simulink model "CtrPlatform_gravity_compensation"  (Simulink 7.9)
settings: Solver=ode3  StartTime=0.0  StopTime=4  FixedStep=Ts  RelTol=1e-3
InitFcn:
  | eval('Config')
StopFcn:
  | eval('tu')
values from neighbouring files (symbols this model uses):
  A = [a1 a2 a3 a4 a5 a6]/180*pi    [Config.m]    (also in CtrPlatformCfg.m)
  a2 = 0    [Config.m]    (also in CtrPlatformCfg.m)
  a3 = 0    [Config.m]    (also in CtrPlatformCfg.m)
  a4 = 0    [Config.m]    (also in CtrPlatformCfg.m)
  a5 = 90    [Config.m]    (also in CtrPlatformCfg.m)
  a6 = 0    [Config.m]    (also in CtrPlatformCfg.m)
  Cen = Cen(:)'    [Config.m]    (also in CtrPlatformCfg.m; DynEulerTest.m = Cen'; EfDynCAD.m = [cen1,cen2,cen3,cen4,cen5,cen6]')
  CurPulseFreq = 0.25*2*pi    (= 1.57079632679)    [Config.m]    (also in CtrPlatformCfg.m)
  Deg2Rad = pi/180    (= 0.0174532925199)    [Config.m]    (also in CtrPlatformCfg.m)
  DisturbSelect = 2    [Config.m]    (also in CtrPlatformCfg.m)
  DynTrjMode = 3    [Config.m]    (also in CtrPlatformCfg.m = 1)
  FbDisturbSelect = 2    [Config.m]    (also in CtrPlatformCfg.m)
  freq = tvel/radius    (= 1)    [Config.m]    (also in CtrPlatformCfg.m)
  Gravity = 9.8    [Config.m]    (also in CtrPlatformCfg.m)
  Ie1 = in1(:)'    [Config.m]    (also in CtrPlatformCfg.m; DynEulerTest.m = in1(:); EfDynCAD.m = in1(:))
  Ie2 = in2(:)'    [Config.m]    (also in CtrPlatformCfg.m; DynEulerTest.m = in2(:); EfDynCAD.m = in2(:))
  Ie3 = in3(:)'    [Config.m]    (also in CtrPlatformCfg.m; DynEulerTest.m = in3(:); EfDynCAD.m = in3(:))
  Ie4 = in4(:)'    [Config.m]    (also in CtrPlatformCfg.m; DynEulerTest.m = in4(:); EfDynCAD.m = in4(:))
  Ie5 = in5(:)'    [Config.m]    (also in CtrPlatformCfg.m; DynEulerTest.m = in5(:); EfDynCAD.m = in5(:))
  Ie6 = in6(:)'    [Config.m]    (also in CtrPlatformCfg.m; DynEulerTest.m = in6(:); EfDynCAD.m = in6(:))
  in1 = [5.2954 -0.2565 -0.6366;-0.2565 4.7000 0.2830;-0.6366 0.2829 5.8635]    [Config.m]    (also in CtrPlatformCfg.m; DynEulerTest.m; EfDynCAD.m = [0.54  -0.01 0.23)
  in2 = [5.8840 0.0072 0.0135;0.0072 6.0178 -0.1907;0.0135 -0.1907 0.3374]    [Config.m]    (also in CtrPlatformCfg.m; DynEulerTest.m; EfDynCAD.m = (R_x*R_z)*in2*(R_x*R_z)')
  in3 = [1.8201 -0.2274 -0.3112;-0.2274 2.2537 -0.1441;-0.3112 -0.1441 1.9485]    [Config.m]    (also in CtrPlatformCfg.m; DynEulerTest.m; EfDynCAD.m = (R_x*R_z)*in3*(R_x*R_z)')
  in4 = [0.0607 -0.0922 0;-0.0922 1.4493 0;0 0 1.4620]    [Config.m]    (also in CtrPlatformCfg.m; DynEulerTest.m = [0.0607 -0.0922 0;-0.0922 1.4493 0;0 0,1.4620]; EfDynCAD.m = (R_y*Rz)*in4*(R_y*Rz)')
  in5 = [0.0191 0.0032 0;0.0032 0.0228 0;0 0 0.0291]    [Config.m]    (also in CtrPlatformCfg.m; DynEulerTest.m; EfDynCAD.m = (R_x*R_y)*in5*(R_x*R_y)')
  in6 = [0.0012 0 0;0 0.0007 0;0 0 0.0007]    [Config.m]    (also in CtrPlatformCfg.m; DynEulerTest.m; EfDynCAD.m = (R_y*Rz)*in6*(R_y*Rz)')
  init_Endx = gd_init(1,4)    [Config.m]    (also in CtrPlatformCfg.m)
  init_Endy = gd_init(2,4)    [Config.m]    (also in CtrPlatformCfg.m)
  init_Endz = gd_init(3,4)    [Config.m]    (also in CtrPlatformCfg.m)
  init_Rot = gd_init(1:3,1:3)    [Config.m]    (also in CtrPlatformCfg.m)
  JntOffset1 = A(1)    [Config.m]    (also in CtrPlatformCfg.m)
  JntOffset2 = A(2)    [Config.m]    (also in CtrPlatformCfg.m)
  JntOffset3 = A(3)    [Config.m]    (also in CtrPlatformCfg.m)
  JntOffset4 = A(4)    [Config.m]    (also in CtrPlatformCfg.m)
  JntOffset5 = A(5)    [Config.m]    (also in CtrPlatformCfg.m)
  JntOffset6 = A(6)    [Config.m]    (also in CtrPlatformCfg.m)
  L = [l1 l2 l3 l4 l5 l6 l7 l8 l9]    [Config.m]    (also in CtrPlatformCfg.m)
  LinePTs2RadpS = 2*pi/(EncRes*Ts)./Gear    [Config.m]    (also in CtrPlatformCfg.m)
  LinePTs2Rpm = 60/(EncRes*Ts)    (= 7.32421875)    [Config.m]    (also in CtrPlatformCfg.m)
  Ma = [ma1 ma2 ma3 ma4 ma5 ma6]    [Config.m]    (also in CtrPlatformCfg.m; DynEulerTest.m = [ma1; ma2; ma3; ma4; ma5; ma6]; EfDynCAD.m = [ma1 ma2 ma3 ma4 ma5 ma6]')
  ma1 = 170.31    [Config.m]    (also in CtrPlatformCfg.m; DynEulerTest.m; EfDynCAD.m = 77.75)
  ma2 = 63.74    [Config.m]    (also in CtrPlatformCfg.m; DynEulerTest.m; EfDynCAD.m = 32.31)
  ma3 = 98.98    [Config.m]    (also in CtrPlatformCfg.m; DynEulerTest.m; EfDynCAD.m = 18.61)
  ma4 = 24.46    [Config.m]    (also in CtrPlatformCfg.m; DynEulerTest.m; EfDynCAD.m = 15.65)
  ma5 = 5.24    [Config.m]    (also in CtrPlatformCfg.m; DynEulerTest.m; EfDynCAD.m = 3.32)
  ma6 = 0.6    [Config.m]    (also in CtrPlatformCfg.m; DynEulerTest.m; EfDynCAD.m)
  PosPulseEnable = 1    [Config.m]    (also in CtrPlatformCfg.m)
  PosVelPulseGain = 500    [Config.m]    (also in CtrPlatformCfg.m)
  Rad2Line = Gear*EncRes/(2*pi)    [Config.m]    (also in CtrPlatformCfg.m)
  Rpm2LinePTs = EncRes*Ts/60    (= 0.136533333333)    [Config.m]    (also in CtrPlatformCfg.m)
  TrajSwitch = 1    [Config.m]    (also in CtrPlatformCfg.m)
  Trq2Cur = Trq2Cur./Cur2Trq    [Config.m]    (also in CtrPlatformCfg.m)
  Ts = 1/FrHz    (= 0.00025)    [Config.m]    (also in CtrPlatformCfg.m)
  Ts_Dyn = Ts    (= 0.00025)    [Config.m]    (also in CtrPlatformCfg.m)
  tvel = 120    [Config.m]    (also in CtrPlatformCfg.m)
  VelLpAxisNum = 1    [Config.m]    (also in CtrPlatformCfg.m)
  VelPulseEnable = 0    [Config.m]    (also in CtrPlatformCfg.m)
  VelPulseGain = 500    [Config.m]    (also in CtrPlatformCfg.m)
  Volt2Trq = Volt2Trq./Trq2Cur    [Config.m]    (also in CtrPlatformCfg.m)
undefined symbols (not defined in the file or in its folder): a1, DiscIntNeverNeededParam, RobotAxis
libraries: simulink x55, mblibv1 x35, powerlib_extras x9, commnoisgen2 x2
(part 4 of 4)

== system CtrPlatform_gravity_compensation/Dynamics/TrjSource/Position Loop Tunning/Axis4 ==
  AbsEnc4 : Constant  Value=JntOffset4
  Discrete Derivative : simulink/Discrete/Discrete Derivative  gainval=1.0  ICPrevScaledInput=0.0  InputProcessing=Inherited  OutMin=[]  OutMax=[]  OutDataType=sfix(16)  OutScaling=2^-10  DoSatur=off
  Discrete-Time Integrator : DiscreteIntegrator  SampleTime=-1  ICPrevOutput=DiscIntNeverNeededParam  ICPrevScaledInput=DiscIntNeverNeededParam
  JntOffset1 : Constant  Value=JntOffset1
  JntOffset2 : Constant  Value=JntOffset2
  JntOffset3 : Constant  Value=JntOffset3
  JntOffset5 : Constant  Value=JntOffset5
  JntOffset6 : Constant  Value=JntOffset6
  LinePTs2RadpS : Gain  Gain=LinePTs2RadpS(4)
  Mux : Mux  Inputs=6
  Mux1 : Mux  Inputs=6
  Mux2 : Mux  Inputs=6
  Sum : Sum  Inputs=++|
  Zero : Constant  Value=0
  JntPos(Rad) : Outport
  JntVel(Rad/s) : Outport  Port=2
  JntAcc(Rad/s2) : Outport  Port=3
  wires:
  LinePTs2RadpS/1 -> Mux1/4, Discrete Derivative/1, Discrete-Time Integrator/1
  Sum/1 -> Mux/4
  JntOffset1/1 -> Mux/1
  [PosVel_Pulse_Dyn] -> LinePTs2RadpS/1
  Discrete Derivative/1 -> Mux2/1
  Discrete-Time Integrator/1 -> Sum/2
  AbsEnc4/1 -> Sum/1
  JntOffset2/1 -> Mux/2
  JntOffset3/1 -> Mux/3
  JntOffset5/1 -> Mux/5
  JntOffset6/1 -> Mux/6
  Zero/1 -> Mux2/6, Mux2/5, Mux2/4, Mux2/3, Mux2/2, Mux1/6, Mux1/1, Mux1/2, Mux1/3, Mux1/5
  Mux/1 -> JntPos(Rad)/1
  Mux1/1 -> JntVel(Rad/s)/1
  Mux2/1 -> JntAcc(Rad/s2)/1

== system CtrPlatform_gravity_compensation/Dynamics/TrjSource/Position Loop Tunning/Axis5 ==
  Discrete Derivative : simulink/Discrete/Discrete Derivative  gainval=1.0  ICPrevScaledInput=0.0  InputProcessing=Inherited  OutMin=[]  OutMax=[]  OutDataType=sfix(16)  OutScaling=2^-10  DoSatur=off
  Discrete-Time Integratr : DiscreteIntegrator  SampleTime=-1  ICPrevOutput=DiscIntNeverNeededParam  ICPrevScaledInput=DiscIntNeverNeededParam
  JntOffset1 : Constant  Value=JntOffset1
  JntOffset2 : Constant  Value=JntOffset2
  JntOffset3 : Constant  Value=JntOffset3
  JntOffset4 : Constant  Value=JntOffset4
  JntOffset5 : Constant  Value=JntOffset5
  JntOffset6 : Constant  Value=JntOffset6
  LinePTs2RadpS : Gain  Gain=LinePTs2RadpS(5)
  Mux : Mux  Inputs=6
  Mux1 : Mux  Inputs=6
  Mux2 : Mux  Inputs=6
  Sum : Sum  Inputs=++|
  Zero : Constant  Value=0
  JntPos(Rad) : Outport
  JntVel(Rad/s) : Outport  Port=2
  JntAcc(Rad/s2) : Outport  Port=3
  wires:
  LinePTs2RadpS/1 -> Mux1/5, Discrete Derivative/1, Discrete-Time Integratr/1
  Discrete Derivative/1 -> Mux2/5
  Sum/1 -> Mux/5
  JntOffset1/1 -> Mux/1
  Mux2/1 -> JntAcc(Rad/s2)/1
  Mux1/1 -> JntVel(Rad/s)/1
  Mux/1 -> JntPos(Rad)/1
  Zero/1 -> Mux2/1, Mux1/1, Mux1/2, Mux1/3, Mux1/4, Mux1/6, Mux2/2, Mux2/3, Mux2/4, Mux2/6
  JntOffset6/1 -> Mux/6
  JntOffset4/1 -> Mux/4
  JntOffset3/1 -> Mux/3
  JntOffset2/1 -> Mux/2
  JntOffset5/1 -> Sum/1
  Discrete-Time Integratr/1 -> Sum/2
  [PosVel_Pulse_Dyn] -> LinePTs2RadpS/1

== system CtrPlatform_gravity_compensation/Dynamics/TrjSource/Position Loop Tunning/Axis6 ==
  Discrete Derivative : simulink/Discrete/Discrete Derivative  gainval=1.0  ICPrevScaledInput=0.0  InputProcessing=Inherited  OutMin=[]  OutMax=[]  OutDataType=sfix(16)  OutScaling=2^-10  DoSatur=off
  Discrete-Time Integrator : DiscreteIntegrator  SampleTime=-1  ICPrevOutput=DiscIntNeverNeededParam  ICPrevScaledInput=DiscIntNeverNeededParam
  JntOffset1 : Constant  Value=JntOffset1
  JntOffset2 : Constant  Value=JntOffset2
  JntOffset3 : Constant  Value=JntOffset3
  JntOffset4 : Constant  Value=JntOffset4
  JntOffset5 : Constant  Value=JntOffset5
  JntOffset6 : Constant  Value=JntOffset6
  LinePTs2RadpS : Gain  Gain=LinePTs2RadpS(6)
  Mux : Mux  Inputs=6
  Mux1 : Mux  Inputs=6
  Mux2 : Mux  Inputs=6
  Sum : Sum  Inputs=++|
  Zero : Constant  Value=0
  JntPos(Rad) : Outport
  JntVel(Rad/s) : Outport  Port=2
  JntAcc(Rad/s2) : Outport  Port=3
  wires:
  LinePTs2RadpS/1 -> Mux1/6, Discrete Derivative/1, Discrete-Time Integrator/1
  Discrete Derivative/1 -> Mux2/6
  JntOffset1/1 -> Mux/1
  Sum/1 -> Mux/6
  [PosVel_Pulse_Dyn] -> LinePTs2RadpS/1
  Discrete-Time Integrator/1 -> Sum/2
  JntOffset6/1 -> Sum/1
  JntOffset2/1 -> Mux/2
  JntOffset3/1 -> Mux/3
  JntOffset4/1 -> Mux/4
  JntOffset5/1 -> Mux/5
  Zero/1 -> Mux2/5, Mux2/4, Mux2/3, Mux2/2, Mux1/5, Mux1/4, Mux1/1, Mux1/2, Mux1/3, Mux2/1
  Mux/1 -> JntPos(Rad)/1
  Mux1/1 -> JntVel(Rad/s)/1
  Mux2/1 -> JntAcc(Rad/s2)/1

== system CtrPlatform_gravity_compensation/Dynamics/TrjSource/Velocity Loop Tunning/Axis1 ==
  Discrete Derivative : simulink/Discrete/Discrete Derivative  gainval=1.0  ICPrevScaledInput=0.0  InputProcessing=Inherited  OutMin=[]  OutMax=[]  OutDataType=sfix(16)  OutScaling=2^-10  DoSatur=off
  Discrete-Time Integrator : DiscreteIntegrator  SampleTime=-1  ICPrevOutput=DiscIntNeverNeededParam  ICPrevScaledInput=DiscIntNeverNeededParam
  JntOffset1 : Constant  Value=JntOffset1  SampleTime=Ts_Dyn
  JntOffset2 : Constant  Value=JntOffset2  SampleTime=Ts_Dyn
  JntOffset3 : Constant  Value=JntOffset3  SampleTime=Ts_Dyn
  JntOffset4 : Constant  Value=JntOffset4  SampleTime=Ts_Dyn
  JntOffset5 : Constant  Value=JntOffset5  SampleTime=Ts_Dyn
  JntOffset6 : Constant  Value=JntOffset6  SampleTime=Ts_Dyn
  LinePTs2RadpS : Gain  Gain=LinePTs2RadpS(1)
  Mux : Mux  Inputs=6
  Mux1 : Mux  Inputs=6
  Mux2 : Mux  Inputs=6
  Sum : Sum  Inputs=++|
  Zero : Constant  Value=0  SampleTime=Ts_Dyn
  JntPos(Rad) : Outport
  JntVel(Rad/s) : Outport  Port=2
  JntAcc(Rad/s2) : Outport  Port=3
  wires:
  [Vel_Pulse_Dyn] -> LinePTs2RadpS/1
  Discrete Derivative/1 -> Mux2/1
  Sum/1 -> Mux/1
  JntOffset1/1 -> Sum/1
  JntOffset2/1 -> Mux/2
  JntOffset3/1 -> Mux/3
  JntOffset4/1 -> Mux/4
  JntOffset5/1 -> Mux/5
  JntOffset6/1 -> Mux/6
  Zero/1 -> Mux2/6, Mux2/5, Mux2/4, Mux2/3, Mux2/2, Mux1/6, Mux1/5, Mux1/4, Mux1/3, Mux1/2
  Mux/1 -> JntPos(Rad)/1
  Mux1/1 -> JntVel(Rad/s)/1
  Mux2/1 -> JntAcc(Rad/s2)/1
  LinePTs2RadpS/1 -> Discrete Derivative/1, Mux1/1, Discrete-Time Integrator/1
  Discrete-Time Integrator/1 -> Sum/2

== system CtrPlatform_gravity_compensation/Dynamics/TrjSource/Velocity Loop Tunning/Axis2 ==
  Discrete Derivative : simulink/Discrete/Discrete Derivative  gainval=1.0  ICPrevScaledInput=0.0  InputProcessing=Inherited  OutMin=[]  OutMax=[]  OutDataType=sfix(16)  OutScaling=2^-10  DoSatur=off
  Discrete-Time Integrator : DiscreteIntegrator  SampleTime=-1  ICPrevOutput=DiscIntNeverNeededParam  ICPrevScaledInput=DiscIntNeverNeededParam
  JntOffset1 : Constant  Value=JntOffset1  SampleTime=Ts_Dyn
  JntOffset2 : Constant  Value=JntOffset2  SampleTime=Ts_Dyn
  JntOffset3 : Constant  Value=JntOffset3  SampleTime=Ts_Dyn
  JntOffset4 : Constant  Value=JntOffset4  SampleTime=Ts_Dyn
  JntOffset5 : Constant  Value=JntOffset5  SampleTime=Ts_Dyn
  JntOffset6 : Constant  Value=JntOffset6  SampleTime=Ts_Dyn
  LinePTs2RadpS : Gain  Gain=LinePTs2RadpS(2)
  Mux : Mux  Inputs=6
  Mux1 : Mux  Inputs=6
  Mux2 : Mux  Inputs=6
  Sum : Sum  Inputs=++|
  Zero : Constant  Value=0  SampleTime=Ts_Dyn
  JntPos(Rad) : Outport
  JntVel(Rad/s) : Outport  Port=2
  JntAcc(Rad/s2) : Outport  Port=3
  wires:
  Mux2/1 -> JntAcc(Rad/s2)/1
  Mux1/1 -> JntVel(Rad/s)/1
  Mux/1 -> JntPos(Rad)/1
  Zero/1 -> Mux2/3, Mux1/4, Mux1/3, Mux1/1, Mux1/5, Mux1/6, Mux2/1, Mux2/4, Mux2/5, Mux2/6
  JntOffset6/1 -> Mux/6
  JntOffset5/1 -> Mux/5
  JntOffset4/1 -> Mux/4
  JntOffset3/1 -> Mux/3
  JntOffset2/1 -> Sum/1
  Discrete-Time Integrator/1 -> Sum/2
  [Vel_Pulse_Dyn] -> LinePTs2RadpS/1
  Sum/1 -> Mux/2
  JntOffset1/1 -> Mux/1
  Discrete Derivative/1 -> Mux2/2
  LinePTs2RadpS/1 -> Discrete-Time Integrator/1, Discrete Derivative/1, Mux1/2

== system CtrPlatform_gravity_compensation/Dynamics/TrjSource/Velocity Loop Tunning/Axis3 ==
  Discrete Derivative : simulink/Discrete/Discrete Derivative  gainval=1.0  ICPrevScaledInput=0.0  InputProcessing=Inherited  OutMin=[]  OutMax=[]  OutDataType=sfix(16)  OutScaling=2^-10  DoSatur=off
  Discrete-Time Integrator : DiscreteIntegrator  SampleTime=-1  ICPrevOutput=DiscIntNeverNeededParam  ICPrevScaledInput=DiscIntNeverNeededParam
  JntOffset1 : Constant  Value=JntOffset1  SampleTime=Ts_Dyn
  JntOffset2 : Constant  Value=JntOffset2  SampleTime=Ts_Dyn
  JntOffset3 : Constant  Value=JntOffset3  SampleTime=Ts_Dyn
  JntOffset4 : Constant  Value=JntOffset4  SampleTime=Ts_Dyn
  JntOffset5 : Constant  Value=JntOffset5  SampleTime=Ts_Dyn
  JntOffset6 : Constant  Value=JntOffset6  SampleTime=Ts_Dyn
  LinePTs2RadpS : Gain  Gain=LinePTs2RadpS(3)
  Mux : Mux  Inputs=6
  Mux1 : Mux  Inputs=6
  Mux2 : Mux  Inputs=6
  Sum : Sum  Inputs=++|
  Zero : Constant  Value=0  SampleTime=Ts_Dyn
  JntPos(Rad) : Outport
  JntVel(Rad/s) : Outport  Port=2
  JntAcc(Rad/s2) : Outport  Port=3
  wires:
  [Vel_Pulse_Dyn] -> LinePTs2RadpS/1
  Discrete-Time Integrator/1 -> Sum/2
  JntOffset3/1 -> Sum/1
  JntOffset2/1 -> Mux/2
  JntOffset4/1 -> Mux/4
  JntOffset5/1 -> Mux/5
  JntOffset6/1 -> Mux/6
  Zero/1 -> Mux2/6, Mux2/5, Mux2/4, Mux2/2, Mux1/6, Mux1/5, Mux1/4, Mux1/2, Mux1/1, Mux2/1
  Mux/1 -> JntPos(Rad)/1
  Mux1/1 -> JntVel(Rad/s)/1
  Mux2/1 -> JntAcc(Rad/s2)/1
  Sum/1 -> Mux/3
  JntOffset1/1 -> Mux/1
  Discrete Derivative/1 -> Mux2/3
  LinePTs2RadpS/1 -> Discrete-Time Integrator/1, Discrete Derivative/1, Mux1/3

== system CtrPlatform_gravity_compensation/Dynamics/TrjSource/Velocity Loop Tunning/Axis4 ==
  AbsEnc4 : Constant  Value=JntOffset4  SampleTime=Ts_Dyn
  Discrete Derivative : simulink/Discrete/Discrete Derivative  gainval=1.0  ICPrevScaledInput=0.0  InputProcessing=Inherited  OutMin=[]  OutMax=[]  OutDataType=sfix(16)  OutScaling=2^-10  DoSatur=off
  Discrete-Time Integrator : DiscreteIntegrator  SampleTime=-1  ICPrevOutput=DiscIntNeverNeededParam  ICPrevScaledInput=DiscIntNeverNeededParam
  JntOffset1 : Constant  Value=JntOffset1  SampleTime=Ts_Dyn
  JntOffset2 : Constant  Value=JntOffset2  SampleTime=Ts_Dyn
  JntOffset3 : Constant  Value=JntOffset3  SampleTime=Ts_Dyn
  JntOffset5 : Constant  Value=JntOffset5  SampleTime=Ts_Dyn
  JntOffset6 : Constant  Value=JntOffset6  SampleTime=Ts_Dyn
  LinePTs2RadpS : Gain  Gain=LinePTs2RadpS(4)
  Mux : Mux  Inputs=6
  Mux1 : Mux  Inputs=6
  Mux2 : Mux  Inputs=6
  Sum : Sum  Inputs=++|
  Zero : Constant  Value=0  SampleTime=Ts_Dyn
  JntPos(Rad) : Outport
  JntVel(Rad/s) : Outport  Port=2
  JntAcc(Rad/s2) : Outport  Port=3
  wires:
  Mux2/1 -> JntAcc(Rad/s2)/1
  Mux1/1 -> JntVel(Rad/s)/1
  Mux/1 -> JntPos(Rad)/1
  Zero/1 -> Mux1/5, Mux1/3, Mux1/2, Mux1/1, Mux1/6, Mux2/2, Mux2/3, Mux2/4, Mux2/5, Mux2/6
  JntOffset6/1 -> Mux/6
  JntOffset5/1 -> Mux/5
  JntOffset3/1 -> Mux/3
  JntOffset2/1 -> Mux/2
  AbsEnc4/1 -> Sum/1
  Discrete-Time Integrator/1 -> Sum/2
  Discrete Derivative/1 -> Mux2/1
  [Vel_Pulse_Dyn] -> LinePTs2RadpS/1
  JntOffset1/1 -> Mux/1
  Sum/1 -> Mux/4
  LinePTs2RadpS/1 -> Discrete-Time Integrator/1, Discrete Derivative/1, Mux1/4

== system CtrPlatform_gravity_compensation/Dynamics/TrjSource/Velocity Loop Tunning/Axis5 ==
  Discrete Derivative : simulink/Discrete/Discrete Derivative  gainval=1.0  ICPrevScaledInput=0.0  InputProcessing=Inherited  OutMin=[]  OutMax=[]  OutDataType=sfix(16)  OutScaling=2^-10  DoSatur=off
  Discrete-Time Integratr : DiscreteIntegrator  SampleTime=-1  ICPrevOutput=DiscIntNeverNeededParam  ICPrevScaledInput=DiscIntNeverNeededParam
  JntOffset1 : Constant  Value=JntOffset1  SampleTime=Ts_Dyn
  JntOffset2 : Constant  Value=JntOffset2  SampleTime=Ts_Dyn
  JntOffset3 : Constant  Value=JntOffset3  SampleTime=Ts_Dyn
  JntOffset4 : Constant  Value=JntOffset4  SampleTime=Ts_Dyn
  JntOffset5 : Constant  Value=JntOffset5  SampleTime=Ts_Dyn
  JntOffset6 : Constant  Value=JntOffset6  SampleTime=Ts_Dyn
  LinePTs2RadpS : Gain  Gain=LinePTs2RadpS(5)
  Mux : Mux  Inputs=6
  Mux1 : Mux  Inputs=6
  Mux2 : Mux  Inputs=6
  Sum : Sum  Inputs=++|
  Zero : Constant  Value=0  SampleTime=Ts_Dyn
  JntPos(Rad) : Outport
  JntVel(Rad/s) : Outport  Port=2
  JntAcc(Rad/s2) : Outport  Port=3
  wires:
  [Vel_Pulse_Dyn] -> LinePTs2RadpS/1
  Discrete-Time Integratr/1 -> Sum/2
  JntOffset5/1 -> Sum/1
  JntOffset2/1 -> Mux/2
  JntOffset3/1 -> Mux/3
  JntOffset4/1 -> Mux/4
  JntOffset6/1 -> Mux/6
  Zero/1 -> Mux2/6, Mux2/4, Mux2/3, Mux2/2, Mux1/6, Mux1/4, Mux1/3, Mux1/2, Mux1/1, Mux2/1
  Mux/1 -> JntPos(Rad)/1
  Mux1/1 -> JntVel(Rad/s)/1
  Mux2/1 -> JntAcc(Rad/s2)/1
  JntOffset1/1 -> Mux/1
  Sum/1 -> Mux/5
  Discrete Derivative/1 -> Mux2/5
  LinePTs2RadpS/1 -> Discrete-Time Integratr/1, Discrete Derivative/1, Mux1/5

== system CtrPlatform_gravity_compensation/Dynamics/TrjSource/Velocity Loop Tunning/Axis6 ==
  Discrete Derivative : simulink/Discrete/Discrete Derivative  gainval=1.0  ICPrevScaledInput=0.0  InputProcessing=Inherited  OutMin=[]  OutMax=[]  OutDataType=sfix(16)  OutScaling=2^-10  DoSatur=off
  Discrete-Time Integrator : DiscreteIntegrator  SampleTime=-1  ICPrevOutput=DiscIntNeverNeededParam  ICPrevScaledInput=DiscIntNeverNeededParam
  JntOffset1 : Constant  Value=JntOffset1
  JntOffset2 : Constant  Value=JntOffset2
  JntOffset3 : Constant  Value=JntOffset3
  JntOffset4 : Constant  Value=JntOffset4
  JntOffset5 : Constant  Value=JntOffset5
  JntOffset6 : Constant  Value=JntOffset6
  LinePTs2RadpS : Gain  Gain=LinePTs2RadpS(6)
  Mux : Mux  Inputs=6
  Mux1 : Mux  Inputs=6
  Mux2 : Mux  Inputs=6
  Sum : Sum  Inputs=++|
  Zero : Constant  Value=0
  JntPos(Rad) : Outport
  JntVel(Rad/s) : Outport  Port=2
  JntAcc(Rad/s2) : Outport  Port=3
  wires:
  Mux2/1 -> JntAcc(Rad/s2)/1
  Mux1/1 -> JntVel(Rad/s)/1
  Mux/1 -> JntPos(Rad)/1
  Zero/1 -> Mux2/2, Mux1/3, Mux1/2, Mux1/1, Mux1/4, Mux1/5, Mux2/1, Mux2/3, Mux2/4, Mux2/5
  JntOffset5/1 -> Mux/5
  JntOffset4/1 -> Mux/4
  JntOffset3/1 -> Mux/3
  JntOffset2/1 -> Mux/2
  JntOffset6/1 -> Sum/1
  Discrete-Time Integrator/1 -> Sum/2
  [Vel_Pulse_Dyn] -> LinePTs2RadpS/1
  Sum/1 -> Mux/6
  JntOffset1/1 -> Mux/1
  Discrete Derivative/1 -> Mux2/6
  LinePTs2RadpS/1 -> Discrete-Time Integrator/1, Discrete Derivative/1, Mux1/6

== matlab function Trajectory Generator/Still/Inverse Kinematic ==
  data: EndPos input double; init_Rot parameter double; Theta output double; L parameter double
function Theta = fcn(EndPos,init_Rot,L)
%#eml
Theta =[0;0; 0; 0; 0; 0];
gd = [init_Rot,EndPos;[0 0 0],1];
[Theta_total,num_total] = inv_kin(gd,L);
%%%%%%%%%%%Need to modify%%%%%%%%%%%%%%%
Theta = Theta_total(:,2);

== matlab function Trajectory Generator/Still/Jacobian ==
  data: Theta input double; Omega output double; EndVel input double; L parameter double
function Omega = fcn(Theta,EndVel,L)
%#eml

Omega = zeros(6,1);
V = [EndVel; 0; 0; 0];   
g = fwd_kin(L,Theta');
Jb = body_Jacobian(L,Theta');
Adg_inv = double(AdjointInv(g));
Omega = double((Jb \ Adg_inv* V)')';

== matlab function Dynamics/M*Acc ==
  data: RefAcc input double; EnTheta input double; M_Acc output double; L parameter double; Cen parameter double; Ma parameter double; Ie1 parameter double; Ie2 parameter double; Ie3 parameter double; Ie4 parameter double; Ie5 parameter double; Ie6 parameter double
function M_Acc = fcn(RefAcc,EnTheta,L,Cen,Ma,Ie1,Ie2,Ie3,Ie4,Ie5,Ie6)
%#eml

M_Acc = zeros(6,1);
M_Acc = M_d(L/1000,EnTheta',Cen,Ma,Ie1,Ie2,Ie3,Ie4,Ie5,Ie6)*RefAcc;

== matlab function Dynamics/C*Omega ==
  data: RefOmega input double; C_Omega output double; EnTheta input double; EnOmega input double; L parameter double; Cen parameter double; Ma parameter double; Ie1 parameter double; Ie2 parameter double; Ie3 parameter double; Ie4 parameter double; Ie5 parameter double; Ie6 parameter double
function C_Omega = fcn(RefOmega,EnTheta,EnOmega,L,Cen,Ma,Ie1,Ie2,Ie3,Ie4,Ie5,Ie6)
%#eml

C_Omega =zeros(6,1);

L=L/1000;
M_dp = zeros(6,6*6);
M_dp(:,1:6) = M_dp1(L,EnTheta',Cen,Ma,Ie1,Ie2,Ie3,Ie4,Ie5,Ie6);
M_dp(:,7:12) = M_dp2(L,EnTheta',Cen,Ma,Ie1,Ie2,Ie3,Ie4,Ie5,Ie6);
M_dp(:,13:18) = M_dp3(L,EnTheta',Cen,Ma,Ie1,Ie2,Ie3,Ie4,Ie5,Ie6);
M_dp(:,19:24)= M_dp4(L,EnTheta',Cen,Ma,Ie1,Ie2,Ie3,Ie4,Ie5,Ie6);
M_dp(:,25:30) = M_dp5(L,EnTheta',Cen,Ma,Ie1,Ie2,Ie3,Ie4,Ie5,Ie6);
M_dp(:,31:36) = M_dp6(L,EnTheta',Cen,Ma,Ie1,Ie2,Ie3,Ie4,Ie5,Ie6);

C = zeros(6,6);

for i=1:6
    for j=1:6
        for k=1:6
                 C(i,j) =C(i,j)+ 0.5*(M_dp(i,(k-1)*6+j)+M_dp(i,(j-1)*6+k)-M_dp(k,(i-1)*6+j))*EnOmega(k);
            
        end
    end
end
C_Omega = C*RefOmega;
% end

== matlab function Dynamics/N ==
  data: EnTheta input double; N output double; L parameter double; Cen parameter double; Ma parameter double; Gravity parameter double
function N = fcn(EnTheta,L,Cen,Ma,Gravity)
%#eml
N=zeros(6,1);
N=N_d(L/1000,EnTheta',Cen,Ma,Gravity);

== matlab function Trajectory Generator/Circle in Descartes Space/Inverse Kinematic ==
  data: EndPos input double; init_Rot parameter double; Theta output double; L parameter double
function Theta = fcn(EndPos,init_Rot,L)
%#eml
Theta =[0;0; 0; 0; 0; 0];
gd = [init_Rot,EndPos;[0 0 0],1];
[Theta_total,num_total] = inv_kin(gd,L);
%%%%%%%%%%%Need to modify%%%%%%%%%%%%%%%
Theta = Theta_total(:,2);

== matlab function Trajectory Generator/Circle in Descartes Space/Jacobian ==
  data: Theta input double; Omega output double; EndVel input double; L parameter double
function Omega = fcn(Theta,EndVel,L)
%#eml

Omega = zeros(6,1);
V = [EndVel; 0; 0; 0];   
g = fwd_kin(L,Theta');
Jb = body_Jacobian(L,Theta');
Adg_inv = double(AdjointInv(g));
Omega = double((Jb \ Adg_inv* V)')';

== matlab function Trajectory Generator/Line in Joint Space/Forward ==
  data: Theta input double; EndPos output double; L parameter double
function EndPos = fcn(Theta,L)
%#eml
gd = fwd_kin(L,Theta');
EndPos = gd(1:3,4);

== matlab function Trajectory Generator/Line in Joint Space/Jacobian ==
  data: Theta input double; Omega input double; EndVel output double; L parameter double
function EndVel = fcn(Theta,Omega,L)
%#eml


EndVW = spat_Jacobian(L,Theta')*Omega;
gd = fwd_kin(L,Theta');
EndW = EndVW(4:6,1);
gd_pos = gd(1:3,4);
EndVel=cross(EndW,gd_pos);
